simulink library "sm_car_lib"  (R2024a)
settings: Solver=VariableStepAuto  StartTime=0.0  StopTime=10.0  RelTol=1e-3
undefined symbols (not defined in the file or in its folder): acc_theta, accel_ramp_rate, circ_out, clr_upr, Control, hp1, hp2, hp3, hp_in_f_ua, hp_in_r_ua, hp_la_out, hp_ua_out, Init, Newton, opc_upr, radius_upr, Raphson, RDF_Rough_Road, rhs_hp, Scene, ShaftF, ShaftR, Vehicle, Visual, X, Y, Z
libraries: sm_lib x117, $bdroot x97, nesl_utility x36, simulink x17, fl_lib x6, sharedtransformsys x3, Brakes_Elements x2, Driver_Gamepad_Xbox x2, Multibody_Parts_Lib x2, sm_car_scene_track_mallory_park_obstacle x2, Testrig_4Post_Inputs x2, Aero_Coefficients x1
(part 1 of 7)
Description:
  | Simscape Vehicle Templates Library
  | 
  | Copyright 2018-2024 The MathWorks, Inc.
settings Model: Creator=mwalker  LastModifiedBy=lnicolet
settings SolverCC: AlgebraicLoopSolver=TrustRegion
settings DataIOCC: ReturnWorkspaceOutputs=off
settings OptimizationCC: ReuseModelBlockBuffer=off
settings DebuggingCC: UnconnectedInputMsg=warning  UnconnectedOutputMsg=warning  UnconnectedLineMsg=warning  ArithmeticOperatorsInVariantConditions=warning
settings ModelReferenceCC: EnableRefExpFcnMdlSchedulingChecks=on
settings SFSimCC: SimUseLocalCustomCode=off  CustomCodeUndefinedFunction=UseInterfaceOnly
settings RTWCC: RTWUseLocalCustomCode=off  GPUComputeCapability=3.5

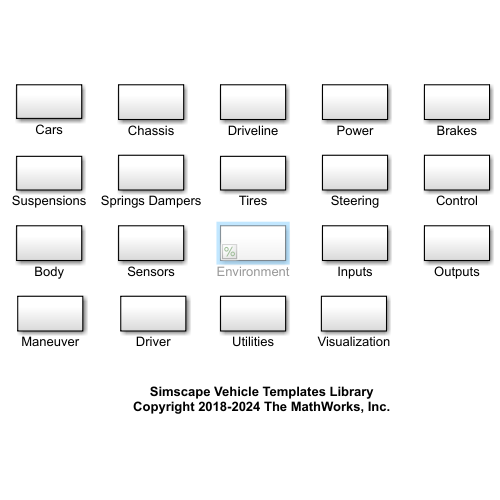
[thumbnail: Simulink's stored preview of the top-level diagram]
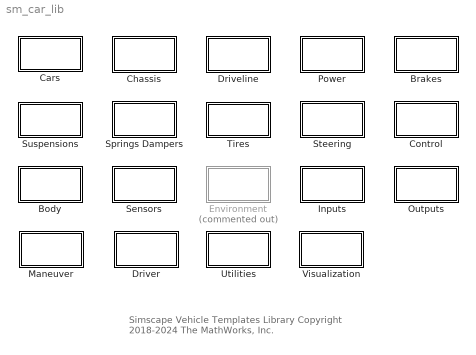
== system sm_car_lib ==
  note: Simscape Vehicle Templates Library
      | Copyright 2018-2024 The MathWorks, Inc.
  Body : Subsystem
  Brakes : Subsystem
  Cars : Subsystem
  Chassis : Subsystem
  Control : Subsystem
  Driveline : Subsystem
  Driver : Subsystem
  Environment : Subsystem  Commented=on
  Inputs : Subsystem
  Maneuver : Subsystem
  Outputs : Subsystem
  Power : Subsystem
  Sensors : Subsystem
  Springs Dampers : Subsystem
  Steering : Subsystem
  Suspensions : Subsystem
  Tires : Subsystem
  Utilities : Subsystem
  Visualization : Subsystem

== system sm_car_lib/Body ==
  Aero : Aero_Coefficients/Aero  CL=Vehicle.Chassis.Aero.CL.Value  CD=Vehicle.Chassis.Aero.CD.Value  rho=Vehicle.Chassis.Aero.rho_air.Value  A=Vehicle.Chassis.Aero.ARef.Value  sCentreOfPressure=Vehicle.Chassis.Aero.sPressureCentre.Value  clr_hp=Visual.hp.clr  opc_hp=Visual.hp.opc  rad_hp=Visual.hp.rad
  Body : Body_Axle2/Body  hp_mount_a1=Chassis.Body.sAxle1.Value  hp_mount_a2=Chassis.Body.sAxle2.Value  hp_mount_power=Chassis.Body.sPower.Value  hp_chassis_cg=Vehicle.Chassis.Body.sCG.Value  hp_mount_hitchf=Chassis.Body.sHitchF.Value  hp_mount_hitchr=Chassis.Body.sHitchR.Value  chassis_mass=Vehicle.Chassis.Body.m.Value  chassis_inertia=Vehicle.Chassis.Body.J.Value  clr_chassis_hp_cg=Visual.hp.clr  opc_chassis_hp_cg=Visual.hp.opc  size_chassis_hp_cg=Visual.hp.rad  BodyGeometry=Vehicle.Chassis.Body.BodyGeometry  Passenger=Vehicle.Chassis.Body.Passenger  BodyLoad=Body.BodyLoad  InitTriggerDropdown=0
  Body to World : Subsystem  mask(Body to World){Init=Init.Chassis, SpecifyPosTarget=on}
      mask prompts: Init "Initial Values"; SpecifyPosTarget "Specify Position Target"
      mask help: Models the connection between the vehicle body and world. Permits 6 degrees of freedom and sets the initial position, orientation, and speed of the vehicle body.
      mask init:
      | initial_aveh = [Init.aChassis.Value(3) Init.aChassis.Value(2) Init.aChassis.Value(1)];
      | rotmat_ypr = sm_car_yawpitchroll_to_rotmat(Init.aChassis.Value(3),Init.aChassis.Value(2),Init.aChassis.Value(1));
      | initial_vveh = rotmat_ypr*(Init.vChassis.Value)';
      | 
      | sptState = get_param(gcb,'SpecifyPosTarget');
      | 
      | set_param([gcb '/Body World Joint'],...
      |         'PxPositionTargetSpecify',sptState,...
      |         'PyPositionTargetSpecify',sptState,...
      |         'PzPositionTargetSpecify',sptState,...
      |         'SphPositionTargetSpecify',sptState,...
      |         'PxVelocityTargetSpecify',sptState,...
      |         'PyVelocityTargetSpecify',sptState,...
      |         'PzVelocityTargetSpecify',sptState...
      |         );
      mask Help: web('sm_car_doc_body_to_world.html')
  Passenger Car : BodyGeometry_Sedan/Sedan  whl_cutout_rad=0.43  whl_base=3.2  thk_top=0.05  thk_side=0.05  car_track=2  offset_ref=BodyGeometry.sOffset.Value  extr_data_emblem_f=Visual.emblem.data*0.2  extr_data_emblem_r=Visual.emblem.data*0.2  clr_body_geo_top=[0.2 0.4 0.6]  opc_body_geo_top=0.3  clr_body_geo_left=[0.2 0.4 0.6]  opc_body_geo_left=0.3  clr_body_geo_right=[0.2 0.4 0.6]  opc_body_geo_right=0.3  clr_emblem_f=[1.0 1.0 1.0]  opc_emblem_f=1.0  clr_emblem_r=[1.0 1.0 1.0]  opc_emblem_r=1.0
  Subsystem : Subsystem

== system sm_car_lib/Brakes ==
  Brakes : Brakes_Axle2/Brakes Axle2  VariantControl=Variant1  LabelModeActiveChoice=PedalAbstract_DiscDisc  Brakes=Vehicle.Brakes  VariantLabel=Vehicle.Brakes.class.Value  InitTriggerDropdown=1
      settings: AttributesFormatString=%<ActiveVariant>
  Brakes 1Axle : Brakes_Axle1/Brakes Axle1  VariantControl=Variant1  LabelModeActiveChoice=None  Brakes=Vehicle.Brakes  VariantLabel=Vehicle.Brakes.class.Value  InitTriggerDropdown=1
      settings: AttributesFormatString=%<ActiveVariant>
  Bus Selector : BusSelector  OutputSignals=Brakes
  Control : $bdroot/Control/Control  popup_brake_control=ABS  trq_ratio_front=1
  DrvBus : $bdroot/Inputs/DrvBus  SystemSampleTime=-1  VariantActivationTime=update diagram  AllowFlexibleInterface=on  Latency=0  AutoFrameSizeCalculation=off
  Pad Rotor : Brakes_Elements/Pad Rotor  d_caliper_piston_f=0.01
  Valve : Brakes_Elements/Valve  area_max=valve_maxA  opening_max=valve_maxO  A_leak=valve_leak  x_0=valve_x0  time_constant=valve_ts  popup_openClose=Open  popup_fault=None
  wires:
  DrvBus/1 -> Brakes/1
  Control/1 -> Bus Selector/1
  Bus Selector/1 -> Brakes/2  "<Brakes>"

== system sm_car_lib/Cars ==
  Control : $bdroot/Control/Control  popup_brake_control=Pedal  trq_ratio_front=1
      settings: AttributesFormatString=%<popup_brake_control>
  Vehicle : Vehicle_Axle2/Vehicle  Tag=PublishSubsystem  VariantControl=NS_Con  Vehicle=Vehicle  Init=Init  SpecifyPosTarget=on  veh_index=1  InitTriggerDropdown=0  mask_image_name=sm_car_vehicle_hamba_IMAGE.png
  wires:
  Control/1 -> Vehicle/2

== system sm_car_lib/Chassis ==
  Bus Selector : BusSelector  OutputSignals=Chassis
  Chassis : Chassis_Axle2/Chassis  Tag=PublishSubsystem  VariantControl=Chassis  Chassis=Vehicle.Chassis  Init=Init  InitTriggerDropdown=1  mask_image_name=sm_car_vehicle_chassis_custom_IMAGE.png  veh_index=1
  Control : $bdroot/Control/Control  popup_brake_control=Pedal  trq_ratio_front=1
      settings: AttributesFormatString=%<popup_brake_control>
  DrvBus : $bdroot/Inputs/DrvBus  SystemSampleTime=-1  VariantActivationTime=update diagram  AllowFlexibleInterface=on  Latency=0  AutoFrameSizeCalculation=off
  Ground : Subsystem
  wires:
  Ground/1(RoadBus) -> Chassis/2
  Control/1 -> Bus Selector/1
  DrvBus/1 -> Chassis/1
  Bus Selector/1 -> Chassis/3  "<Chassis>"

== system sm_car_lib/Control ==
  Brake Control : Subsystem  Variant=on  VariantControlMode=label  VariantControl=Variant1  LabelModeActiveChoice=Pedal  mask{popup_brake_control=Pedal, abs_tire_radiusF=0.35, abs_tire_radiusR=0.35}
      mask prompts: popup_brake_control "Control Type"; abs_tire_radiusF "Tire Radius Front (m)"; abs_tire_radiusR "Tire Radius Rear (m)"
      mask init:
      | set_param(gcb,'LabelModeActiveChoice',get_param(gcb,'popup_brake_control'));
      settings: AttributesFormatString=%<ActiveVariant>
      mask TypeOptions popup_brake_control: Pedal | Pressure | ABS
      mask Display: disp(' ');
  Control : Subsystem  mask{popup_brake_control=Pedal, trq_ratio_front=1}
      mask prompts: popup_brake_control "Brake Control"; trq_ratio_front "Ratio of Torque on Front Wheels (0-1)"
      mask init:
      | if(popup_brake_control == 1)
      |     set_param([gcb '/Brake Control'],'popup_brake_control','Pedal');
      | elseif(popup_brake_control == 2)
      |     set_param([gcb '/Brake Control'],'popup_brake_control','Pressure');
      | elseif(popup_brake_control == 3)
      |     set_param([gcb '/Brake Control'],'popup_brake_control','ABS');
      | end
      settings: AttributesFormatString=%<popup_brake_control>
      mask TypeOptions popup_brake_control: Pedal | Pressure | ABS
      mask TypeOptions trq_ratio_front: Power Control/trq_ratio_front
  Driveline Control : Subsystem
  Power Control : Subsystem  mask{trq_max=1600, trq_ratio_front=1, trq_rate_up=300, trq_rate_down=-5000}
      mask prompts: trq_max "Max Torque Request"; trq_ratio_front "Ratio of Torque on Front Wheels (0-1)"; trq_rate_up "Torque Rate Limit Up (N*m/s)"; trq_rate_down "Torque Rate Limit Down (N*m/s)"
  Steer : Subsystem  mask{Steer=Control.Default.Steer}
      mask prompts: Steer "Steer (structure)"
  Steer Axle3 : Subsystem  mask{nSteerA2=Control.Default.steer_ratio_axle2, nSteerA3=Control.Default.steer_ratio_axle3}
      mask prompts: nSteerA2 "Axle 2 Steer Ratio"; nSteerA3 "Axle 3 Steer Ratio"
  Valve Control : Subsystem
  VehBus : $bdroot/Outputs/VehBus  SystemSampleTime=-1  VariantActivationTime=update diagram  AllowFlexibleInterface=on  Latency=0  AutoFrameSizeCalculation=off
  wires:
  VehBus/1 -> Brake Control/2("VehBus ")

== system sm_car_lib/Driveline ==
  Differential : Differential_Systems/Differential  VariantControl=Variant1  Differential=Driveline.DifferentialF  VariantLabel=Driveline.DifferentialF.class.Value  InitTriggerDropdown=1
      settings: AttributesFormatString=%<ActiveVariant>
  Driveline : Driveline_Axle2/Driveline Axle2  VariantControl=Shaft  LabelModeActiveChoice=A1_A2_A1Diff_A2Diff  Driveline=Vehicle.Powertrain.Driveline  VariantLabel=Vehicle.Powertrain.Driveline.class.Value  InitTriggerDropdown=1
      settings: AttributesFormatString=%<ActiveVariant>
  Driveline 1Axle : Driveline_Axle1/Driveline Axle1  VariantControl=Shaft  LabelModeActiveChoice=None  Driveline=Vehicle.Powertrain.Driveline  VariantLabel=Vehicle.Powertrain.Driveline.class.Value  InitTriggerDropdown=1
      settings: AttributesFormatString=%<ActiveVariant>
  Driveline Control : $bdroot/Control/Driveline Control  SystemSampleTime=-1  VariantActivationTime=update diagram  AllowFlexibleInterface=on  Latency=0  AutoFrameSizeCalculation=off
  Driveline Shafts Terminator : Subsystem
  Driveshaft : Driveshaft_ShaftsAll/Driveshaft  VariantControl=Variant1  popup_leftRight=Right  Driveshaft=Vehicle.Powertrain.Driveline.DriveshaftFR  VariantLabel=Vehicle.Powertrain.Driveline.DriveshaftFR.class.Value  InitTriggerDropdown=1
      settings: AttributesFormatString=%<ActiveVariant>
  Shaft : Differential_Components/Shaft  popup_leftRight=Left  shaft_m=3.5  len_shaft=0.4  clr_shaft=Visual.Driveshaft.clr  opc_shaft=Visual.part.opc  rad_shaft=Visual.Driveshaft.rad
  wires:
  Driveline Control/1 -> Driveline/1
  connections:
  Driveline/LConn4 -- Driveline Shafts Terminator/RConn1

== system sm_car_lib/Driver ==
  Driver Inputs Xbox : Driver_Gamepad_Xbox/Gamepad Xbox/Driver Inputs Xbox  SystemSampleTime=-1  VariantActivationTime=update diagram  AllowFlexibleInterface=on  Latency=0  AutoFrameSizeCalculation=off
  Gamepad Xbox : Driver_Gamepad_Xbox/Gamepad Xbox  SystemSampleTime=-1  VariantActivationTime=update diagram  AllowFlexibleInterface=on  Latency=0  AutoFrameSizeCalculation=off
  Long Lat Stanley : Driver_Long_Lat_Stanley/Long Lat Stanley  Driver=Driver
  Open Loop : Driver_Open_Loop/Open Loop  Maneuver=Maneuver

== system sm_car_lib/Environment ==
  note: Full Scene Variant Selection
      | Add new scenes here by pasting
      | a library link as a new variant.
      | Scene selection done
      | in CarWorld Config
  note: Scene Elements
  CarWorldConfig : Subsystem  mask(Environment){UseLocalSolver=off, LocalSolverChoice=Backward Euler, LocalSolverSampleTime=0.005, DoFixedCost=off, MaxNonlinIter=3, popup_scene=Plane Grid, popup_gravity=Constant, GravityVector=[0 0 -9.80665]}
      mask prompts: UseLocalSolver "Use Local Solver"; LocalSolverChoice "Solver Type:"; LocalSolverSampleTime "Sample time"; DoFixedCost "Use fixed-cost"; MaxNonlinIter "Number of iterations"; popup_scene "Scene"; popup_gravity "Gravity Model"; GravityVector "Gravity Vector [x y z] (m/s^2)"
      mask help: World frame, driving surface, gravity, and solver settings.
      mask init:
      | if(LocalSolverChoice == 1)
      |     solverChoice = 'NE_BACKWARD_EULER_ADVANCER';
      | elseif(LocalSolverChoice == 2)
      |     solverChoice = 'NE_TRAPEZOIDAL_ADVANCER';
      | elseif(LocalSolverChoice == 3)
      |     solverChoice = 'NE_PARTITIONING_ADVANCER';
      | end
      | set_param([gcb '/Solver Configuration'],'LocalSolverChoice',solverChoice)
      | 
      | tempblkscenename = strrep(get_param(gcb,'popup_scene'),' ','_');
      | set_param([gcb '/Scene'],'LabelModeActiveChoice',tempblkscenename);
      | gravityModel = get_param(gcb,'popup_gravity');
      | if(strcmpi(gravityModel,'constant'))
      |     set_param([gcb '/Mechanism Configuration'],'LabelModeActiveChoice','ConstantGravity');
      | elseif(strcmpi(gravityModel,'ramp x and y components'))
      |     set_param([gcb '/Mechanism Configuration'],'LabelModeActiveChoice','VariableGravityXY');
      | end
      | clear tempblkscenename
      settings: AttributesFormatString=|
      | %<popup_scene>
      | Local Solver: %<UseLocalSolver>
      mask TypeOptions UseLocalSolver:
      | Solver
      | Configuration/UseLocalSolver
      mask Callback UseLocalSolver:
      | maskObj = Simulink.Mask.get(gcb);
      | 
      | samTM_h = maskObj.getParameter('LocalSolverSampleTime');
      | slvCH_h = maskObj.getParameter('LocalSolverChoice');
      | fixCT_h = maskObj.getParameter('DoFixedCost');
      | 
      | temp_useLSstate = get_param(gcb,'UseLocalSolver');
      | samTM_h.Enabled = temp_useLSstate;
      | slvCH_h.Enabled = temp_useLSstate;
      | fixCT_h.Enabled = temp_useLSstate;
      | 
      | clear maskObj
      | clear samTM_h slvCH_h fixCT_h
      | clear temp_useLSstate
      mask TypeOptions LocalSolverChoice: Backward Euler | Trapezoidal Rule | Partitioning
      mask TypeOptions LocalSolverSampleTime:
      | Solver
      | Configuration/LocalSolverSampleTime
      mask TypeOptions DoFixedCost:
      | Solver
      | Configuration/DoFixedCost
      mask Callback DoFixedCost:
      | maskObj = Simulink.Mask.get(gcb);
      | 
      | numIT_h = maskObj.getParameter('MaxNonlinIter');
      | 
      | temp_doFixCoststate = get_param(gcb,'DoFixedCost');
      | numIT_h.Enabled = temp_doFixCoststate;
      | 
      | clear maskObj numIT_h temp_doFixCoststate
      mask TypeOptions MaxNonlinIter:
      | Solver
      | Configuration/MaxNonlinIter
      mask TypeOptions popup_scene: Plane Grid | Road Two Lane | Double Lane Change | Double Lane Change ISO3888 | Ice Patch | RDF Rough Road | Rough Road Z Only | CRG Rough Road | RDF Plateau | Plateau Z Only | CRG Plateau | Track Mallory Park | Track Mallory Park Obstacle | MCity | CRG Hockenheim | CRG Hockenheim F | CRG Kyalami | CRG Kyalami F | CRG Mallory Park | CRG Mallory Park F | CRG Nurburgring N | CRG Nurburgring N F | CRG Pikes Peak | CRG Suzuka | CRG Suzuka F | CRG Custom | CRG Custom F | Skidpad | Constant Radius | Testrig 4 Post
      mask TypeOptions popup_gravity: Constant | Ramp x and y components
      mask Display: disp('Wld')
  Check 2x2 : Subsystem  mask{square_lwh=[0.01 1 1]}
      mask prompts: square_lwh "Size [l w h] (m)"
  Cone : Subsystem  mask(Cone){height=1, baseThickness=0.1, baseWidth=0.6, coneBaseDiameter=0.4, coneTopDiameter=0.1, reflectiveStripHeight=0.5, coneColor=[1 0.6 0], reflectiveStripColor=[0.75 0.75 0.75]}
      mask prompts: height "Height (m)"; baseThickness "Base Thickness (m)"; baseWidth "Base Width (m)"; coneBaseDiameter "Cone Base Diameter (m)"; coneTopDiameter "Cone Top Diameter (m)"; reflectiveStripHeight "Reflective Strip Height (m)"; coneColor "Cone Color [r g b]"; reflectiveStripColor "Reflective Strip Color [r g b]"
      mask help:
      | This block models a traffic cone. The block comprises an octagonal base with a conical upper.
      |
      | Port B corresponds to the center point of the bottom surface of the base with the z-axis aligned with the conical axis.
      mask init:
      | coneBaseHeight = 0.5 * (height - baseThickness - reflectiveStripHeight);
      | 
      | coneHeight = height - baseThickness;
      | 
      | coneBaseRadius = 0.5 * coneBaseDiameter;
      | coneTopRadius2 = 0.5 * coneTopDiameter;
      | 
      | coneRadDiff = coneBaseRadius - coneTopRadius2;
      | 
      | coneBaseRadius2 = coneBaseRadius - coneBaseHeight * coneRadDiff / coneHeight;
      | 
      | coneBaseCrossSection = [0 0; 
      |                         coneBaseRadius 0;
      |                         coneBaseRadius2 coneBaseHeight;
      |                         0 coneBaseHeight];
      | 
      | coneTopHeight = coneBaseHeight;
      | coneTopRadius1 = coneTopRadius2 + coneTopHeight * coneRadDiff / coneHeight;
      |                       
      | reflectiveStripCrossSection = [0 0;
      |                                coneBaseRadius2 0;
      |                                coneTopRadius1 reflectiveStripHeight;
      |                                0 reflectiveStripHeight];
      |                              
      | coneTopCrossSection = [0 0;
      |                        coneTopRadius1 0;
      |                        coneTopRadius2 coneTopHeight;
      |                        0 coneTopHeight];
      mask DialogControl Tab1 Prompt: Dimensions
      mask DialogControl Tab2 Prompt: Material Properties
      mask Display:
      | image(imread(fullfile(matlabroot,'toolbox','physmod','sm','smdemos','vehicle_slalom','images','sm_vehicle_slalom_cone.png')));
      | port_label('lconn',1,'B');
  Cones Double Lane Change : Subsystem  mask{lane_width=3.3, lane_separation=4.1, start_lane_a=173.8, A1_to_A5=12.5, A_to_B_x=12.7, B1_to_B5=12.3, B_to_C_x=12.7, C1_to_C5=12, height=0.6, baseThickness=0.04, baseWidth=0.5, coneBaseDiameter=0.24, coneTopDiameter=0.06, reflectiveStripHeight=0.3, coneColor=[248 78 25]/255, reflectiveStripColor=[0.75 0.75 0.75]}
      mask prompts: lane_width "Lane Width (m)"; lane_separation "Lane Lateral Separation (m)"; start_lane_a "Distance to start Lane A (m)"; A1_to_A5 "Distance Cone 1 to 5 (m) Lane A"; A_to_B_x "Distance Lane A to Lane B (m)"; B1_to_B5 "Distance Cone 1 to 5 (m) Lane B"; B_to_C_x "Distance Lane B to Lane C (m)"; C1_to_C5 "Distance Cone 1 to 5 (m) Lane C"; height "Height (m)"; baseThickness "Base Thickness (m)"; baseWidth "Base Width (m)"; coneBaseDiameter "Cone Base Diameter (m)"; coneTopDiameter "Cone Top Diameter (m)"; reflectiveStripHeight "Reflective Strip Height (m)"; coneColor "Cone Color [RGB]"; reflectiveStripColor "Reflective Strip Color [RGB]"
      mask DialogControl cont_placement Prompt: Placement
      mask DialogControl cont_appearance Prompt: Appearance
  Dashes : Subsystem  mask{dash_pitch=7.5, num_dashes=4, dash_l=3, dash_h=2, dash_w=0.15, thickness_base=4, dash_clr=[1 1 1], dash_opc=1}
      mask prompts: dash_pitch "Distance between dash centers (m)"; num_dashes "Number of dashes"; dash_l "Dash length (m)"; dash_h "Dash height (m)"; dash_w "Dash width (m)"; thickness_base "Height base of solid (m)"; dash_clr "Color [RGB]"; dash_opc "Opacity (0-1)"
      mask init:
      | dash_extr_data = Extr_Data_Dashes(dash_pitch,num_dashes,dash_l,dash_h,thickness_base);
  Finish Line : Subsystem  mask{post_h=6, post_r=0.5, line_w=18, post_clr=[0.8 0.0 0.2], post_opc=1, offset_xyz=[0 0 0], offset_yaw=0, offset_pitch=0, offset_roll=0}
      mask prompts: post_h "Post Height (m)"; post_r "Post Radius (m)"; line_w "Post Separation (m)"; post_clr "Post Color [R G B] (0-1)"; post_opc "Post Opacity (0-1)"; offset_xyz "Line Offset [x y z] (m)"; offset_yaw "Line Orientation yaw (rad)"; offset_pitch "Line Orientation pitch (rad)"; offset_roll "Line Orientation roll (rad)"
  Grid : Subsystem  mask{grid_x=400, grid_y=400, grid_z=0.02, grid_line_width=0.08, grid_num_sq_x=10, grid_num_sq_y=17, grid_clr=[1 1 1], grid_opc=1}
      mask prompts: grid_x "Length (m) (Global x)"; grid_y "Width (m) (Global y)"; grid_z "Depth (m) (Global z)"; grid_line_width "Line width (m)"; grid_num_sq_x "Number of squares in x"; grid_num_sq_y "Number of squares in y"; grid_clr "Color [RGB]"; grid_opc "Opacity (0-1)"
      mask init:
      | % Derived parameters - for two perpendicular grids with num_sq-by-1 holes
      | % **Note, not num_sq_x by num_sq_y holes - better render speed with
      | % separate meshes for x and y.
      | 
      | hole_lx = (grid_x-(grid_line_width*(grid_num_sq_x+1)))/grid_num_sq_x;
      | hole_wx = (grid_y-(grid_line_width*(1+1)))/1;
      | 
      | hole_ly = (grid_y-(grid_line_width*(grid_num_sq_y+1)))/grid_num_sq_y;
      | hole_wy = (grid_x-(grid_line_width*(1+1)))/1;
  Override : Subsystem  Variant=on  VariantControlMode=label  VariantControl=Variant1  LabelModeActiveChoice=None  mask{popup_override_type=None}
      mask prompts: popup_override_type "Override Type"
      mask init:
      | set_param(gcb,'LabelModeActiveChoice',strrep(get_param(gcb,'popup_override_type'),' ','_'));
      mask TypeOptions popup_override_type: None | Track Mallory Park Obstacle
      mask Display: disp(' ');
  Patch Rectangle : Subsystem  mask{gp_l=400, gp_w=400, gp_h=0.01, gp_clr=[0.8000 0.8000 0.8000], gp_opc=1}
      mask prompts: gp_l "Length (m) (Global  x)"; gp_w "Width (m) (Global  y)"; gp_h "Depth (m) (Global z)"; gp_clr "Color [R G B]"; gp_opc "Opacity (0-1)"
  RDF Polyline : Subsystem  mask{road_extr_data_L=RDF_Rough_Road.Road.extr_data_L, road_extr_data_R=RDF_Rough_Road.Road.extr_data_R, road_profile_sep=RDF_Rough_Road.Road.profile_separation, road_w=RDF_Rough_Road.Road.w, road_x=RDF_Rough_Road.Road.x, road_z=RDF_Rough_Road.Road.z, road_yaw=RDF_Rough_Road.Road.yaw, road_clr=RDF_Rough_Road.Road.clr, road_opc=RDF_Rough_Road.Road.opc}
      mask prompts: road_extr_data_L "Road Profile Left [x y] (m)"; road_extr_data_R "Road Profile Right [x y] (m)"; road_profile_sep "Profile Separation (m)"; road_w "Width (m)"; road_x "Offset x (m)"; road_z "Offset z (m)"; road_yaw "Offset yaw (rad)"; road_clr "Color [R G B]"; road_opc "Opacity (0-1)"
  Road Surface Profile : Subsystem  Variant=on  VariantControlMode=label  LabelModeActiveChoice=None
      settings: AttributesFormatString=%<LabelModeActiveChoice>
      mask Display: disp(' ')
  Road Surface Profile Axle3 : Subsystem  Variant=on  VariantControlMode=label  LabelModeActiveChoice=None
      settings: AttributesFormatString=%<LabelModeActiveChoice>
      mask Display: disp(' ')
  Road z vs x Left Right : Subsystem  VariantControl=Variant  mask{dist_x_l=flipud(Scene.RDF_Plateau.Road.extr_data_L(45:end,1)), height_z_l=flipud(Scene.RDF_Plateau.Road.extr_data_L(45:end,2)), dist_x_r=flipud(Scene.RDF_Plateau.Road.extr_data_R(45:end,1)), height_z_r=flipud(Scene.RDF_Plateau.Road.extr_data_R(45:end,2))}
      mask prompts: dist_x_l "Distance Vector Left [x] (m)"; height_z_l "Height Vector Left [z] (m)"; dist_x_r "Distance Vector Right [x] (m)"; height_z_r "Height Vector Right [z] (m)"
      mask init:
      | pitch_l = atan2(circshift(height_z_l,-2)-circshift(height_z_l,2),circshift(dist_x_l,-2)-circshift(dist_x_l,2));
      | pitch_l(1:2) = pitch_l(3);
      | pitch_l(end-1:end) = pitch_l(end-2);
      | 
      | pitch_r = atan2(circshift(height_z_r,-2)-circshift(height_z_r,2),circshift(dist_x_r,-2)-circshift(dist_x_r,2));
      | pitch_r(1:2) = pitch_r(3);
      | pitch_r(end-1:end) = pitch_r(end-2);
  Road z vs x Left Right Axle3 : Subsystem  VariantControl=Variant  mask{dist_x_l=flipud(Scene.RDF_Plateau.Road.extr_data_L(45:end,1)), height_z_l=flipud(Scene.RDF_Plateau.Road.extr_data_L(45:end,2)), dist_x_r=flipud(Scene.RDF_Plateau.Road.extr_data_R(45:end,1)), height_z_r=flipud(Scene.RDF_Plateau.Road.extr_data_R(45:end,2))}
      mask prompts: dist_x_l "Distance Vector Left [x] (m)"; height_z_l "Height Vector Left [z] (m)"; dist_x_r "Distance Vector Right [x] (m)"; height_z_r "Height Vector Right [z] (m)"
      mask init: same as sm_car_lib/Environment/Road z vs x Left Right
  "Road z vs x " : Subsystem  VariantControl=Variant  mask{dist_x=flipud(Scene.RDF_Plateau.Road.extr_data_L(45:end,1)), height_z=flipud(Scene.RDF_Plateau.Road.extr_data_L(45:end,2))}
      mask prompts: dist_x "Distance vector [x] (m)"; height_z "Height vector [z] (m)"
      mask init:
      | pitch_rd = atan2(circshift(height_z,-2)-circshift(height_z,2),circshift(dist_x,-2)-circshift(dist_x,2));
      | pitch_rd(1:2) = pitch_rd(3);
      | pitch_rd(end-1:end) = pitch_rd(end-2);
  Road z vs x Axle3 : Subsystem  VariantControl=Variant  mask{dist_x=flipud(Scene.RDF_Plateau.Road.extr_data_L(45:end,1)), height_z=flipud(Scene.RDF_Plateau.Road.extr_data_L(45:end,2))}
      mask prompts: dist_x "Distance vector [x] (m)"; height_z "Height vector [z] (m)"
      mask init:
      | pitch_rd = atan2(circshift(height_z,-2)-circshift(height_z,2),circshift(dist_x,-2)-circshift(dist_x,2));
      | pitch_rd(1:2) = pitch_rd(3);
      | pitch_rd(end-1:end) = pitch_rd(end-2);
  STL Geometry : Subsystem  mask{stl_file='Bar1_Default_sldprt.STL', stl_units='m', stl_clr=[0.8000 0.8000 0.8000], stl_opc=1, stl_x=0, stl_y=0, stl_z=0, stl_yaw=0, stl_pitch=0, stl_roll=0}
      mask prompts: stl_file "CAD File"; stl_units "Units"; stl_clr "Color [R G B]"; stl_opc "Opacity (0-1)"; stl_x "Offset x (m)"; stl_y "Offset y (m)"; stl_z "Offset z (m)"; stl_yaw "Offset yaw (rad)"; stl_pitch "Offset pitch (rad)"; stl_roll "Offset roll (rad)"
      mask init:
      | set_param([gcb '/Geometry'],'ExtGeomFileName',stl_file);
      | set_param([gcb '/Geometry'],'ExtGeomFileUnits',stl_units);
  Scene : Subsystem  Variant=on  VariantControlMode=label  LabelModeActiveChoice=Road_Two_Lane
      settings: AttributesFormatString=%<LabelModeActiveChoice>
  Solver Configuration : nesl_utility/Solver Configuration  PhysicalDomain=network_engine_domain  SubClassName=solver  LeftPortType=input  RightPortType=generic  Tones=[]  Harmonics=[]  SimulateNoise=off  Profile=off  UseLocalSampling=off  EnableSwitchedLinearOptims=on  FrequencyDomain=off  UseCCode=off  RelTol=0.001  AbsTol=1e-06  MinStep=1e-09  ToWorkspace=off  RevertToSquareIcSolve=off  NumHomotopyIterations=100  PhasorMode=off  PhasorModeNumHarmonics=1  ConsistencySolver=NEWTON_FTOL  IndexReductionMethod=DerivativeReplacement  DoDC=off  ResidualTolerance=1e-09  ConsistencyTolSource=GLOBAL  ConsistencyAbsTol=0.001  ConsistencyRelTol=0.001  ConsistencyTolFactor=0.001  UseLocalSolver=on  LocalSolverChoice=NE_BACKWARD_EULER_ADVANCER  ResolveIndetEquations=on  FunctionEvalNumThread=1  LocalSolverSampleTime=0.001  DoFixedCost=on  MaxNonlinIter=3  MaxModeIter=2  ComputeImpulses=off  ImpulseIterations=2  LinearAlgebra=auto  LinearAlgebraNumThread=0  EquationFormulation=NE_TIME_EF  DelaysMemoryBudget=1024  AutomaticFiltering=on  FilteringTimeConstant=0.001  PartitionStorageMethod=AS_NEEDED  PartitionMemoryBudget=1024  PartitionMethod=FAST  MultibodyUseLocalSolver=off  MultibodyLocalSolverChoice=ODE1  MultibodyLocalSolverSampleTime=0.001
  Stripe Ring : Subsystem  mask{circ_d=circ_out.d, circ_a1=circ_out.ang1, circ_a2=circ_out.ang2, circ_w=circ_out.w, circ_h=circ_out.h, circ_clr=circ_out.clr, circ_opc=circ_out.opc}
      mask prompts: circ_d "Circle Diameter (m)"; circ_a1 "Start Angle (deg)"; circ_a2 "Finish Angle (deg)"; circ_w "Stripe Width (m)"; circ_h "Stripe Height (m)"; circ_clr "Color [RGB]"; circ_opc "Opacity (0-1)"
      mask init:
      | xy_data_circ = Extr_Data_Ring(...
      |     circ_d/2+circ_w/2,circ_d/2-circ_w/2,circ_a1, circ_a2);
  Track Extrusion : Subsystem  mask{track_ctrline=[sin(0:0.1:(2*pi-0.1))' cos(0:0.1:(2*pi-0.1))' cos(0:0.1:(2*pi-0.1))']*10, track_w=2, track_h=0.1, track_x=0, track_y=0, track_z=0, track_yaw=0, track_clr=[0.8000 0.8000 0.8000], track_opc=1}
      mask prompts: track_ctrline "Centerline profile [x y] (m)"; track_w "Width (m)"; track_h "Height (m)"; track_x "Offset x (m)"; track_y "Offset y (m)"; track_z "Offset z (m)"; track_yaw "Offset yaw (rad)"; track_clr "Color [R G B]"; track_opc "Opacity (0-1)"
      mask init:
      | track_extr_data = sm_car_road_track_extrusion(track_ctrline,track_w);

== system sm_car_lib/Inputs ==
  Control Bus : Subsystem
  Control Bus Axle3 : Subsystem
  DrvBus : Subsystem
  Road Bus : Subsystem
  Terminator : Terminator
  wires:
  DrvBus/1(Out1) -> Terminator/1

== system sm_car_lib/Maneuver ==
  Check : Subsystem  mask{stop_speed=0.1, start_check_time=5, max_speed=0.4, start_check_time_max_speed=20000, lat_dev_threshold=8, start_check_time_ld=10000, start_check_time_end_lap=10000}
      mask TypeOptions stop_speed: Stop Threshold/Value
      mask TypeOptions start_check_time: Start Checking/Time
      mask TypeOptions max_speed: Max Speed Threshold/Value
      mask TypeOptions start_check_time_max_speed: Start Checking Max Speed/Time
      mask TypeOptions lat_dev_threshold: Lateral Deviation Threshold/Value
      mask TypeOptions start_check_time_ld: Start Checking Lat Dev/Time
      mask TypeOptions start_check_time_end_lap: Start Checking End Lap/Time
      mask DialogControl text_quantity Prompt: Quantity
      mask DialogControl text_start_check Prompt: Start Check (sec)
      mask DialogControl text_final_speed Prompt: Final Speed (m/s)
      mask DialogControl text_max_speed Prompt: Max Speed (m/s)
      mask DialogControl text_max_lat_dev Prompt: Max Lateral Offset (m)
      mask DialogControl text_end_lap_1 Prompt: End Lap 1
  Maneuver : Maneuver_Get_Pose/Maneuver  Maneuver=Maneuver  popup_window=No

== system sm_car_lib/Outputs ==
  Terminator : Terminator
  VehBus : Subsystem
  wires:
  VehBus/1(VehBus) -> Terminator/1

== system sm_car_lib/Power ==
  Power : Power_Systems/Power  VariantControl=Variant1  LabelModeActiveChoice=Ideal_A1_A2  Power=Vehicle.Powertrain.Power  VariantLabel=Vehicle.Powertrain.Power.class.Value  InitTriggerDropdown=1
      settings: AttributesFormatString=%<ActiveVariant>

== system sm_car_lib/Sensors ==
  Body Sensor : Subsystem  mask{offset_body_sensor=Vehicle.Chassis.Body.sCG.Value}
      mask prompts: offset_body_sensor "Sensor Frame Offset [x y z] (m)"
  Body Sensor Empty : Subsystem  mask{offset_body_sensor=Vehicle.Chassis.Body.sCG.Value}
      mask prompts: offset_body_sensor "Sensor Frame Offset [x y z] (m)"

== system sm_car_lib/Springs Dampers ==
  Dampers : Dampers_Axle2/Dampers Axle2  VariantControl=Variant1  LabelModeActiveChoice=Independent  Damper=Vehicle.Chassis.Damper  VariantLabel=Vehicle.Chassis.Damper.class.Value  InitTriggerDropdown=1
      settings: AttributesFormatString=%<ActiveVariant>
  Dampers 1Axle : Dampers_Axle1/Dampers Axle1  VariantControl=Variant1  LabelModeActiveChoice=Independent  Damper=Vehicle.Chassis.Damper  VariantLabel=Vehicle.Chassis.Damper.class.Value  InitTriggerDropdown=1
      settings: AttributesFormatString=%<ActiveVariant>
  Springs : Springs_Axle2/Springs Axle2  VariantControl=Variant1  LabelModeActiveChoice=Independent  Spring=Vehicle.Chassis.Spring  VariantLabel=Vehicle.Chassis.Spring.class.Value  InitTriggerDropdown=1
      settings: AttributesFormatString=%<ActiveVariant>
  Springs 1Axle : Springs_Axle1/Springs Axle1  VariantControl=Variant1  LabelModeActiveChoice=Independent  Spring=Vehicle.Chassis.Spring  VariantLabel=Vehicle.Chassis.Spring.class.Value  InitTriggerDropdown=1
      settings: AttributesFormatString=%<ActiveVariant>

== system sm_car_lib/Steering ==
  Steer : Steer_Rack_System/Steer  VariantControl=Steer  Steer=Vehicle.Chassis.SuspF.Steer  VariantLabel=Vehicle.Chassis.SuspF.Steer.class.Value  InitTriggerDropdown=1
      settings: AttributesFormatString=%<ActiveVariant>
  Steer Input : $bdroot/Inputs/DrvBus/Steer Input  popup_steer_input=Sequence
  Steer1 : $bdroot/Inputs/Control Bus/Susp  SystemSampleTime=-1  VariantActivationTime=update diagram  AllowFlexibleInterface=on  Latency=0  AutoFrameSizeCalculation=off
  wires:
  Steer Input/1 -> Steer/1
  Steer1/1 -> Steer/2

== system sm_car_lib/Suspensions ==
  DrvBus : $bdroot/Inputs/DrvBus  SystemSampleTime=-1  VariantActivationTime=update diagram  AllowFlexibleInterface=on  Latency=0  AutoFrameSizeCalculation=off
  Linkage : Linkage_Systems/Linkage  VariantControl=Variant1  LabelModeActiveChoice=DoubleWishbone  popup_leftRight=Left  Linkage=Vehicle.Chassis.SuspA1.Linkage  InitLinkage=Init.Axle1  VariantLabel=Vehicle.Chassis.SuspA1.Linkage.class.Value  InitTriggerDropdown=1
      settings: AttributesFormatString=%<ActiveVariant>
  Subsystem : $bdroot/Inputs/Control Bus/Susp  SystemSampleTime=-1  VariantActivationTime=update diagram  AllowFlexibleInterface=on  Latency=0  AutoFrameSizeCalculation=off
  Suspension and Steering : Suspension_Systems/Suspension and Steering  VariantControl=Variant1  LabelModeActiveChoice=Linkage  Susp=Vehicle.Chassis.SuspA1  Init=Init.Axle1  VariantLabel=Vehicle.Chassis.SuspA1.class.Value  InitTriggerDropdown=1
  Terminator : Terminator
  Wheel Measurements : Subsystem
  wires:
  Subsystem/1 -> Suspension and Steering/1
  Subsystem/2 -> Terminator/1
  DrvBus/1 -> Suspension and Steering/2

== system sm_car_lib/Tires ==
  note: Set to 0.6 for low friction
      | surface if using Delft Tyre
  Bus Creator : BusCreator  Inputs=4
  Bus Selector : BusSelector  OutputSignals=L1
  Constant1 : Constant
  Constant2 : Constant
  Ground : Subsystem
  Ground1 : Subsystem
  Mu Scaling by Position : Subsystem  mask{muFL_out=1, muFR_out=1, muRL_out=1, muRR_out=1, muFL_in=1, muFR_in=1, muRL_in=1, muRR_in=1, intvX_FL_start=100-40, intvX_FR_start=100-40, intvX_RL_start=100-40, intvX_RR_start=100-40, intvX_FL_end=130-40, intvX_FR_end=130-40, intvX_RL_end=130-40, intvX_RR_end=130-40, intvY_FL_start=-30, intvY_FR_start=-30, intvY_RL_start=-30, intvY_RR_start=-30, intvY_FL_end=0, intvY_FR_end=0, intvY_RL_end=0, intvY_RR_end=0}
      mask TypeOptions muFL_out: muL1 out/Value
      mask TypeOptions muFR_out: muR1 out/Value
      mask TypeOptions muRL_out: muL2 out/Value
      mask TypeOptions muRR_out: muR2 out/Value
      mask TypeOptions muFL_in: muL 1in/Value
      mask TypeOptions muFR_in: muR1 in/Value
      mask TypeOptions muRL_in: muL2 in/Value
      mask TypeOptions muRR_in: muR2 in/Value
      mask TypeOptions intvX_FL_start: Interval Test L1x/lowlimit
      mask TypeOptions intvX_FR_start: Interval Test R1x/lowlimit
      mask TypeOptions intvX_RL_start: Interval Test L2x/lowlimit
      mask TypeOptions intvX_RR_start: Interval Test R2x/lowlimit
      mask TypeOptions intvX_FL_end: Interval Test L1x/uplimit
      mask TypeOptions intvX_FR_end: Interval Test R1x/uplimit
      mask TypeOptions intvX_RL_end: Interval Test L2x/uplimit
      mask TypeOptions intvX_RR_end: Interval Test R2x/uplimit
      mask TypeOptions intvY_FL_start: Interval Test L1y/lowlimit
      mask TypeOptions intvY_FR_start: Interval Test R1y/lowlimit
      mask TypeOptions intvY_RL_start: Interval Test L2y/lowlimit
      mask TypeOptions intvY_RR_start: Interval Test R2y/lowlimit
      mask TypeOptions intvY_FL_end: Interval Test L1y/uplimit
      mask TypeOptions intvY_FR_end: Interval Test R1y/uplimit
      mask TypeOptions intvY_RL_end: Interval Test L2y/uplimit
      mask TypeOptions intvY_RR_end: Interval Test R2y/uplimit
      mask DialogControl text_whl Prompt: Wheel
      mask DialogControl text_FL Prompt: FL
      mask DialogControl text_FR Prompt: FR
      mask DialogControl text_RL Prompt: RL
      mask DialogControl text_RR Prompt: RR
      mask DialogControl text_mu Prompt: mu
      mask DialogControl text_mu_intv Prompt: mu intv
      mask DialogControl text_x_start Prompt: X Start (m)
      mask DialogControl text_x_end Prompt: X End (m)
      mask DialogControl text_y_start Prompt: Y Start (m)
      mask DialogControl text_y_end Prompt: Y End (m)
  None : $bdroot/Environment/Road Surface Profile/None  SystemSampleTime=-1  VariantControl=None  VariantActivationTime=update diagram  AllowFlexibleInterface=on  Latency=0  AutoFrameSizeCalculation=off
  None1 : $bdroot/Environment/Road Surface Profile Axle3/None  SystemSampleTime=-1  VariantControl=None  VariantActivationTime=update diagram  AllowFlexibleInterface=on  Latency=0  AutoFrameSizeCalculation=off
  Scaling factors 4 : Subsystem  mask{LKX=1, LKY=1, LKYC=1, LTR=1, LKZC=1}
      mask prompts: LKX "longitudinal slip stiffness"; LKY "cornering stiffness"; LKYC "camber stiffness"; LTR "pneumatic trail"; LKZC "camber torque stiffness"
  Sensor Wheel Frame : Subsystem
  Tire Body : TireBody_Models/Tire Body  LabelModeActiveChoice=Parameterized  popup_leftRight=Right  TireBody=Vehicle.Chassis.TireF.TireBody  VariantLabel=Vehicle.Chassis.TireF.TireBody.class.Value  InitTriggerDropdown=1
      settings: AttributesFormatString=%<LabelModeActiveChoice>
  Tire Body temp hold : Subsystem  mask{radius=0.4225, rim_radius=0.3048, width=0.235, rim_width=0.235*0.1, mass=10, rim_mass=0, tire_inertia=[1 2], rim_inertia=[0 0], popup_leftRight=Left, clr_tyre=[0.5 0.5 0.5], opc_tyre=1.0, clr_rim=[0.8 0.8 0.8], opc_rim=0.5}
      mask prompts: popup_leftRight "Left/Right"
      mask init:
      | % Change rim location if wheel is on right side
      | if (popup_leftRight == 1)
      |     rhs_tire = 1;
      | elseif(popup_leftRight == 2)
      |     rhs_tire = -1;
      | end
      | 
      | Imat = [tire_inertia(1)+rim_inertia(1) 0 0; 0 tire_inertia(1)+rim_inertia(1) 0; 0 0 tire_inertia(2)+rim_inertia(2)];
      mask TypeOptions popup_leftRight: Left | Right
      mask TypeOptions clr_tyre: Tire/GraphicDiffuseColor
      mask TypeOptions opc_tyre: Tire/GraphicOpacity
      mask TypeOptions clr_rim: Rim/GraphicDiffuseColor
      mask TypeOptions opc_rim: Rim/GraphicOpacity
      mask DialogControl cont_tyre Prompt: Tire Geometry
      mask DialogControl group_tyre_dim Prompt: Dimensions
      mask DialogControl text_tyre_tire Prompt: Tyre
      mask DialogControl text_tyre_rim Prompt: Rim
      mask DialogControl text_tyre_dim_radius Prompt: Radius (m)
      mask DialogControl text_tyre_dim_width Prompt: Width (m)
      mask DialogControl text_tyre_mass Prompt: Mass (kg)
      mask DialogControl text_tyre_inertia Prompt: Inertia [Ixx Iyy]
      mask DialogControl cont_tyre_vis Prompt: Visualization
      mask DialogControl text_vis_tyre_clr Prompt: Color [RGB]
      mask DialogControl text_vis_tyre_opc Prompt: Opacity (0-1)
      mask DialogControl text_vis_tyre_tyre Prompt: Tyre
      mask DialogControl text_vis_tyre_rim Prompt: Rim
  Tire Models : Tire_Models/Tire Models  Tag=PublishSubsystem  VariantControl=Variant1  LabelModeActiveChoice=MFMbody  popup_leftRight=Right  tir_index=1  Tire=Vehicle.Chassis.TireF  VariantLabel=Vehicle.Chassis.TireF.class.Value  InitTriggerDropdown=1
      settings: AttributesFormatString=%<ActiveVariant>
  wires:
  Bus Selector/1 -> Tire Models/1  "<L1>"
  Bus Creator/1 -> ?  "RdBus"
  Scaling factors 4/1(scaling) -> Ground/6(TyreScaling RR), Ground/5(TyreScaling RL), Ground/3(TyreScaling FL), Ground/4(TyreScaling FR)
  Constant1/1 -> Scaling factors 4/1(muX)
  Constant2/1 -> Scaling factors 4/2(muY)
  None/1 -> Ground/1(gz)  "gz"
  Ground/1(L1) -> Bus Creator/1
  Ground/2(R1) -> Bus Creator/2
  Ground/3(L2) -> Bus Creator/3
  Ground/4(R2) -> Bus Creator/4
  None/2 -> Ground/2(uvec)
  None1/2 -> Ground1/2(uvec)
  None1/1 -> Ground1/1(gz)
  Mu Scaling by Position/1(L1) -> Ground1/3(TyreScaling L1)
  Mu Scaling by Position/2(R1) -> Ground1/4(TyreScaling R1)
  Mu Scaling by Position/3(L2) -> Ground1/5(TyreScaling L2)
  Mu Scaling by Position/4(R2) -> Ground1/6(TyreScaling R2)
  Mu Scaling by Position/5(L3) -> Ground1/7(TyreScaling L3)
  Mu Scaling by Position/6(R3) -> Ground1/8(TyreScaling R3)

== system sm_car_lib/Utilities ==
  Camera Frames : Camera_Frame_Definitions/Camera Frames  Camera=Camera  popup_dolly_camera=Off
  Cylinder Between Two Points : Subsystem  mask(Cylinder between two points){hp_b=hp_la_out.*rhs_hp, hp_f=hp_ua_out.*rhs_hp, Mass=0, clr_solid=clr_upr*0+[0.2 0.4 0.6], opc_solid=opc_upr*0.5, rad_solid=radius_upr*1.5}
      mask prompts: hp_b "Hardpoint at B [xyz] (m)"; hp_f "Hardpoint at F [xyz] (m)"; Mass "Mass (kg)"; clr_solid "Color [RGB]"; opc_solid "Opacity (0-1)"; rad_solid "Radius (m)"
      mask help: Models a cylinder parameterized by its end points.
      mask TypeOptions Mass: Solid/Mass
      mask TypeOptions clr_solid: Solid/GraphicDiffuseColor
      mask TypeOptions opc_solid: Solid/GraphicOpacity
      mask TypeOptions rad_solid: Solid/CylinderRadius
      mask DialogControl cont_vis Prompt: Visualization
      mask Display: image('sm_car_cylinder_two_points.png')
  Primitive Bushing : Subsystem
      mask Display: image('sm_car_primitive_bushing.png');
  Primitive Gimbal : Subsystem
      mask Display: image('sm_car_primitive_gimbal.png')
  Q to Z-Y-X Extrinsic : Subsystem
  Revolute Align Axis Three Points : Subsystem  mask(Revolute Joint 3 Points){popup_leftRight=Left, hp_1=[0 0 0], hp_2=[1 0 1], hp_3=[0 1 1]}
      mask prompts: popup_leftRight "Left/Right"; hp_1 "Hardpoint 1 [xyz] (m)"; hp_2 "Hardpoint 2 [xyz] (m)"; hp_3 "Hardpoint 3 [xyz] (m)"
      mask help:
      | Revolute Joint with degree of freedom normal to 3 hardpoints.
      |
      | Positive z-axis will point along cross (HP1 -> HP3, HP1->HP2).
      mask init:
      | % Set parameter for mirroring (+y or -y)
      | if(popup_leftRight == 1)
      |     rhs_susp = 1;
      | elseif(popup_leftRight == 2)
      |     rhs_susp = -1;
      | end
      | rhs_hp = [1 rhs_susp 1];
      | 
      | if(popup_leftRight == 1)
      |     set_param([gcb '/Transform Align Axis B'],'popup_f_axis','+Z');
      |     set_param([gcb '/Transform Align Axis F'],'popup_f_axis','+Z');
      | elseif(popup_leftRight == 2)
      |     set_param([gcb '/Transform Align Axis B'],'popup_f_axis','-Z');
      |     set_param([gcb '/Transform Align Axis F'],'popup_f_axis','-Z');
      | end
      mask TypeOptions popup_leftRight: Left | Right
      mask Display: image('sm_car_variant_revolute.png')
  Rotational Simscape Intf : Subsystem
  Terminator : Subsystem
  Transform Align Axis Three Points : Subsystem  mask(Transform Align Axis Three Points){pt1=hp1, pt2=hp2, pt3=hp3, popup_f_axis=+Z}
      mask prompts: pt1 "Point 1 [xyz] (m)"; pt2 "Point 2 [xyz] (m)"; pt3 "Point 3 [xyz] (m)"; popup_f_axis "Axis of F Frame to Aim at Target"
      mask help: Transforms a frame to aim a selected axis along a normal to a plane defined by 3 points. All points must be defined relative to the same reference frame. Normal to the plane is defined as cross (HP1 -> HP3, HP1->HP2).
      mask init:
      | switch popup_f_axis
      |     case 1, vec = [ 1  0  0];
      |     case 2, vec = [ 0  1  0];
      |     case 3, vec = [ 0  0  1];
      |     case 4, vec = [-1  0  0];
      |     case 5, vec = [ 0 -1  0];
      |     case 6, vec = [ 0  0 -1];
      | end
      | 
      | % Unit vectors 
      | uvec1 = (pt3-pt1)/norm(pt3-pt1);
      | uvec2 = (pt2-pt1)/norm(pt2-pt1);
      | 
      | nvec = cross(uvec1,uvec2);
      | unvec = nvec/norm(nvec);
      | 
      | % Force nvec to point along +z
      | %if(unvec(3)<0)
      | %    unvec = -unvec;
      | %end
      | rotaxis = cross(vec,unvec);
      | 
      | if (norm(rotaxis)==0)
      |     if (sum(uvec1==0)==3 || sum(uvec2==0)==3)  % hps collocated
      |         rotangle = 0; 
      |     elseif ((sum(uvec1+uvec2)==0) ...  % vectors antiparallel    
      |             || (sum(vec+unvec))==0)    % vec and unvec antiparallel
      |         rotangle = pi;
      |         rotaxis = circshift(vec,1);
      |     else                       % vectors parallel
      |         rotangle = 0;          
      |     end
      | else
      |     rotangle = acos(dot(vec,unvec));
      |     %rotangle = acos(dot(vec,(hp_t-hp_b)/norm((hp_t-hp_b))))
      | end
      mask TypeOptions popup_f_axis: +X | +Y | +Z | -X | -Y | -Z
      mask Display: image('sm_car_transform_align_axis_three_points.png')
  Transform Align Axis Two Points : Subsystem  mask(Transform Align Axis Two Points){hp_b=hp1, hp_t=hp2, popup_f_axis=-Z}
      mask prompts: hp_b "Location of B [xyz] (m)"; hp_t "Target for Frame Axis [xyz] (m)"; popup_f_axis "Axis of F Frame to Aim at Target"
      mask help: Transforms a frame to aim a selected axis at a target point. Both points must be defined relative to the same reference frame.
      mask init:
      | switch popup_f_axis
      |     case 1, vec = [ 1  0  0];
      |     case 2, vec = [ 0  1  0];
      |     case 3, vec = [ 0  0  1];
      |     case 4, vec = [-1  0  0];
      |     case 5, vec = [ 0 -1  0];
      |     case 6, vec = [ 0  0 -1];
      | end
      | 
      | uvec_bt = (hp_t-hp_b)/norm(hp_t-hp_b);
      | rotaxis = cross(vec,uvec_bt);
      | 
      | if (norm(rotaxis)==0)
      |     if (uvec_bt==0)            % hps collocated
      |         rotangle = 0; 
      |     elseif ((uvec_bt+vec)==0)  % vectors antiparallel    
      |         rotangle = pi;
      |         rotaxis = circshift(vec,1);
      |     else                       % vectors parallel
      |         rotangle = 0;          
      |     end
      | else
      |     rotangle = acos(dot(vec,uvec_bt));
      |     %rotangle = acos(dot(vec,(hp_t-hp_b)/norm((hp_t-hp_b))))
      | end
      mask TypeOptions popup_f_axis: +X | +Y | +Z | -X | -Y | -Z
      mask Display: image('sm_car_transform_align_axis_two_points.png')
  Translational Simscape Intf : Subsystem
  Universal Two HP : Subsystem  mask{popup_leftRight=Left, hp_f=hp_in_f_ua, hp_r=hp_in_r_ua}
      mask prompts: popup_leftRight "Left/Right"; hp_f "HP Front [xyz] (m)"; hp_r "HP Rear [xyz] (m)"
      mask init:
      | if(popup_leftRight == 1)
      |     rhs_y = 1;
      | elseif(popup_leftRight == 2)
      |     rhs_y = -1;
      | end
      | 
      | rhs_hp = [1 rhs_y 1];
      mask TypeOptions popup_leftRight: Left | Right
      mask Display: image('sm_car_variant_universal.png');

== system sm_car_lib/Visualization ==
  XY Plot : Vehicle_Visualization/XY Plot  SystemSampleTime=-1  VariantActivationTime=update diagram  AllowFlexibleInterface=on  Latency=0  AutoFrameSizeCalculation=off
